simulink model "VSG_loadPR1116"  (R2015a)
settings: Solver=ode23tb  StartTime=0.0  StopTime=2  MaxStep=1e-4  MinStep=1e-7  RelTol=1e-7
InitFcn:
  | fs=1/10e3;
  | gTs=1/10e3;
libraries: powerlib x18, powerlib_meascontrol x6
settings Model: Creator=ewei  LastModifiedBy=GenkiShoo
settings DebuggingCC: UnderspecifiedInitializationDetection=Classic  MergeDetectMultiDrivingBlocksExec=none  SolverPrmCheckMsg=warning  StateNameClashWarn=warning

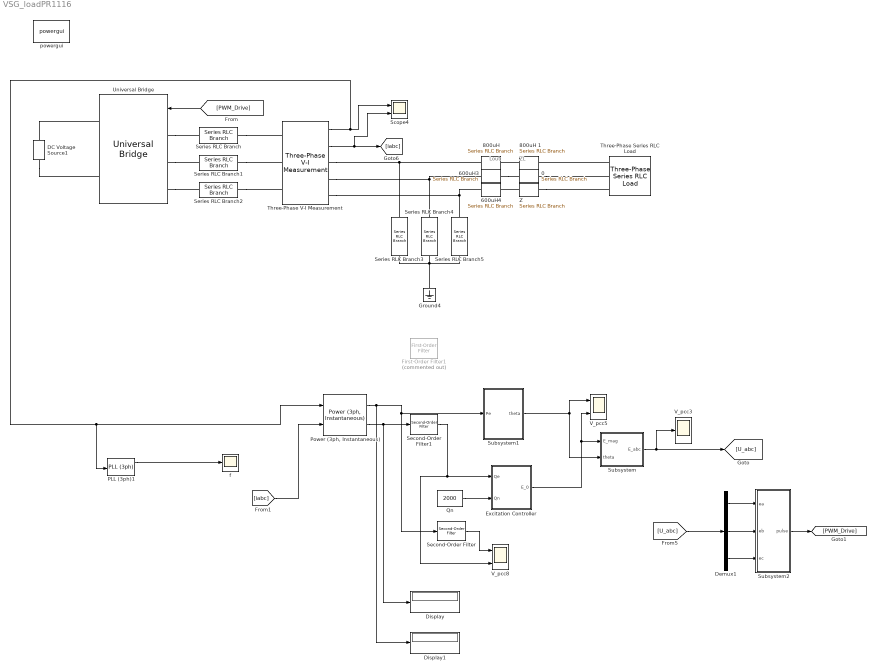
== system VSG_loadPR1116 ==
  note: ZL
  note: Lout
  0 : powerlib/Elements/Series RLC Branch  LConnTagsString=__new0  RConnTagsString=__new0  BranchType=R  Resistance=0.077+0.017i  Inductance=6e-3  SetiL0=off  InitialCurrent=0  Capacitance=[]  Setx0=off  InitialVoltage=0  Measurements=None
  600uH3 : powerlib/Elements/Series RLC Branch  LConnTagsString=__new0  RConnTagsString=__new0  BranchType=L  Resistance=0.001  Inductance=6e-3  SetiL0=off  InitialCurrent=0  Capacitance=[]  Setx0=off  InitialVoltage=0  Measurements=None
  600uH4 : powerlib/Elements/Series RLC Branch  LConnTagsString=__new0  RConnTagsString=__new0  BranchType=L  Resistance=0.001  Inductance=6e-3  SetiL0=off  InitialCurrent=0  Capacitance=[]  Setx0=off  InitialVoltage=0  Measurements=None
  "800uH " : powerlib/Elements/Series RLC Branch  LConnTagsString=__new0  RConnTagsString=__new0  BranchType=L  Resistance=0.001  Inductance=6e-3  SetiL0=off  InitialCurrent=0  Capacitance=[]  Setx0=off  InitialVoltage=0  Measurements=None
  800uH 1 : powerlib/Elements/Series RLC Branch  LConnTagsString=__new0  RConnTagsString=__new0  BranchType=R  Resistance=0.077+0.017i  Inductance=6e-3  SetiL0=off  InitialCurrent=0  Capacitance=[]  Setx0=off  InitialVoltage=0  Measurements=None
  DC Voltage Source1 : powerlib/Electrical Sources/DC Voltage Source  Amplitude=1000  Measurements=None
  Demux1 : Demux  Outputs=3
  Display : Display
  Display1 : Display
  Excitation Controller : Subsystem  mask{K=1/6000, U0=311}
  First-Order Filter1 : powerlib_meascontrol/Filters/First-Order Filter  Commented=on  FilterType=Lowpass  Tc=10e-3  Ts=0  Initialize=on  Vac_Init=[0, 0, 52]  Vdc_Init=0  PlotResponse=off  FreqRange="[0,  200,  1]"
  Ground4 : powerlib/Elements/Ground  LConnTagsString=a
  PLL (3ph)1 : powerlib_meascontrol/PLL/PLL (3ph)  Fmin=45  Par_Init=[0, 50]  ParK=[180, 3200, 1]  TcD=1e-4  MaxRateChangeFreq=12  FilterCutOffFreq=25  Ts=0  AGC=on
  "Power (3ph, Instantaneous)" : powerlib_meascontrol/Measurements/Power (3ph, Instantaneous)
  Qn : Constant  Value=2000
  Scope4 : Scope  NumInputPorts=2
      settings: YMin=-550~-150  YMax=550~125  SaveName=ScopeData8
  Second-Order Filter : powerlib_meascontrol/Filters/Second-Order Filter  FilterType=Lowpass  Fo=20  Zeta=0.707  Ts=0  Initialize=off  Vac_Init="[0,  0,  60]"  Vdc_Init=0  PlotResponse=off  FreqRange=[0, 500, 1]
  Second-Order Filter1 : powerlib_meascontrol/Filters/Second-Order Filter  FilterType=Lowpass  Fo=20  Zeta=0.707  Ts=0  Initialize=off  Vac_Init="[0,  0,  60]"  Vdc_Init=0  PlotResponse=off  FreqRange=[0, 500, 1]
  Series RLC Branch : powerlib/Elements/Series RLC Branch  LConnTagsString=__new0  RConnTagsString=__new0  BranchType=RL  Resistance=0.1  Inductance=2e-3  SetiL0=off  InitialCurrent=0  Capacitance=1e-6  Setx0=off  InitialVoltage=0  Measurements=None
  Series RLC Branch1 : powerlib/Elements/Series RLC Branch  LConnTagsString=__new0  RConnTagsString=__new0  BranchType=RL  Resistance=0.1  Inductance=2e-3  SetiL0=off  InitialCurrent=0  Capacitance=1e-6  Setx0=off  InitialVoltage=0  Measurements=None
  Series RLC Branch2 : powerlib/Elements/Series RLC Branch  LConnTagsString=__new0  RConnTagsString=__new0  BranchType=RL  Resistance=0.1  Inductance=2e-3  SetiL0=off  InitialCurrent=0  Capacitance=1e-6  Setx0=off  InitialVoltage=0  Measurements=None
  Series RLC Branch3 : powerlib/Elements/Series RLC Branch  LConnTagsString=__new0  RConnTagsString=__new0  BranchType=RC  Resistance=4  Inductance=1e-3  SetiL0=off  InitialCurrent=0  Capacitance=40e-6  Setx0=off  InitialVoltage=0  Measurements=None
  Series RLC Branch4 : powerlib/Elements/Series RLC Branch  LConnTagsString=__new0  RConnTagsString=__new0  BranchType=RC  Resistance=4  Inductance=1e-3  SetiL0=off  InitialCurrent=0  Capacitance=40e-6  Setx0=off  InitialVoltage=0  Measurements=None
  Series RLC Branch5 : powerlib/Elements/Series RLC Branch  LConnTagsString=__new0  RConnTagsString=__new0  BranchType=RC  Resistance=4  Inductance=1e-3  SetiL0=off  InitialCurrent=0  Capacitance=40e-6  Setx0=off  InitialVoltage=0  Measurements=None
  Subsystem : Subsystem
  Subsystem1 : Subsystem  mask{w0=314.15, R=1/10000, Tj=400, Kd=0, P0=20000}
      mask DialogControl parameter Prompt: parameter
  Subsystem2 : Subsystem
  Three-Phase Series RLC Load : powerlib/Elements/Three-Phase Series RLC Load  LConnTagsString=A|B|C  Configuration=Y (grounded)  NominalVoltage=380  NominalFrequency=50  ActivePower=17500  InductivePower=8000  CapacitivePower=0  Measurements=Branch voltages and currents  LoadType=constant Z
  Three-Phase V-I Measurement : powerlib/Measurements/Three-Phase V-I Measurement  VoltageMeasurement=phase-to-ground  SetLabelV=off  LabelV=Vabc  Vpu=off  VpuLL=off  CurrentMeasurement=yes  SetLabelI=off  LabelI=Iabc  Ipu=off  Pbase=100e6  Vbase=500e3  OutputType=Complex  PhasorSimulation=off  PSBequivalent=0
  Universal Bridge : powerlib/Power Electronics/Universal Bridge  Arms=3  SnubberResistance=1e5  SnubberCapacitance=inf  Device=IGBT / Diodes  Ron=1e-3  Lon=0  ForwardVoltages="[  0  0  ]"  ForwardVoltage=0  GTOparameters=[ 10e-6 , 20e-6 ]  IGBTparameters=[ 1e-6 , 2e-6 ]  Measurements=None  Measurements_2=None  converterType=Rectifier
  V_pcc3 : Scope
      settings: TimeRange=0.06000000000000001  YMin=-350  YMax=300
  V_pcc5 : Scope  NumInputPorts=2
      settings: TimeRange=2  YMin=120~312.291  YMax=126.5~312.291  SaveName=ScopeData7
  V_pcc8 : Scope  NumInputPorts=2
      settings: YMin=12600~6875  YMax=13050~7350  SaveName=ScopeData9
  Z : powerlib/Elements/Series RLC Branch  LConnTagsString=__new0  RConnTagsString=__new0  BranchType=R  Resistance=0.077+0.017i  Inductance=6e-3  SetiL0=off  InitialCurrent=0  Capacitance=[]  Setx0=off  InitialVoltage=0  Measurements=None
  f : Scope
      settings: YMin=50.259  YMax=50.272  SaveName=ScopeData10
  powergui : powerlib/powergui  Priority=1  SimulationMode=Discrete  SolverType=Tustin  SampleTime=5e-6  frequency=60  SPID=on  DisableSnubberDevices=off  DisableRonSwitches=off  DisableVfSwitches=off  SwTol=0  DisplayEquations=off  Interpol=off  methode=off  Ts=0  FunctionMessages=off  echomessages=off  HookPort=off  EnableUseOfTLC=off  x0status=blocks  frequencyindice=0  Pbase=100e6  ErrMax=1e-4  Iterations=50  UnitsV=kV  UnitsW=MW  buscounter=0  RestoreLinks=warning  ResistiveCurrentMeasurement=off  Frange=[0:2:500]  Ylog=off  Xlog=on  ShowGrid=off  save=off  variable=ZData  structure=0  ZoomFFT=off  StartTime=0.0  cycles=1  DisplayStyle=1  fundamental=60  FreqAxis=off  MaxFrequency=1000  frequencyindicesteady=1  RmsSteady=1  display=off
  wires:
  [PWM_Drive] -> Universal Bridge/1
  Qn/1 -> Excitation Controller/2(Qn)
  Excitation Controller/1(E_0) -> Subsystem/1(E_mag), V_pcc5/2
  Subsystem/1(E_abc) -> V_pcc3/1, [U_abc]
  Three-Phase V-I Measurement/2 -> Scope4/2, [iabc]
  Subsystem1/1(theta) -> Subsystem/2(theta), V_pcc5/1
  Subsystem2/1(pulse) -> [PWM_Drive]
  Demux1/1 -> Subsystem2/1(ea)
  [U_abc] -> Demux1/1
  Demux1/2 -> Subsystem2/2(eb)
  Demux1/3 -> Subsystem2/3(ec)
  "Power (3ph, Instantaneous)"/1 -> Display1/1, Second-Order Filter/1, Subsystem1/1(Pe)
  "Power (3ph, Instantaneous)"/2 -> Display/1, Second-Order Filter1/1
  PLL (3ph)1/1 -> f/1
  Three-Phase V-I Measurement/1 -> "Power (3ph, Instantaneous)"/1, PLL (3ph)1/1, Scope4/1
  [iabc] -> "Power (3ph, Instantaneous)"/2
  Second-Order Filter/1 -> V_pcc8/1
  Second-Order Filter1/1 -> V_pcc8/2, Excitation Controller/1(Qe)
  connections:
  Three-Phase V-I Measurement/RConn3 -- Series RLC Branch5/RConn1 -- 600uH4/LConn1
  Three-Phase V-I Measurement/RConn2 -- Series RLC Branch4/RConn1 -- 600uH3/LConn1
  Three-Phase V-I Measurement/RConn1 -- "800uH "/LConn1 -- Series RLC Branch3/RConn1
  DC Voltage Source1/LConn1 -- Universal Bridge/RConn2
  Series RLC Branch/RConn1 -- Three-Phase V-I Measurement/LConn1
  Series RLC Branch1/RConn1 -- Three-Phase V-I Measurement/LConn2
  DC Voltage Source1/RConn1 -- Universal Bridge/RConn1
  Series RLC Branch2/RConn1 -- Three-Phase V-I Measurement/LConn3
  Series RLC Branch3/LConn1 -- Ground4/LConn1 -- Series RLC Branch5/LConn1 -- Series RLC Branch4/LConn1
  800uH 1/LConn1 -- "800uH "/RConn1
  600uH3/RConn1 -- 0/LConn1
  Z/LConn1 -- 600uH4/RConn1
  Universal Bridge/LConn2 -- Series RLC Branch1/LConn1
  Universal Bridge/LConn3 -- Series RLC Branch2/LConn1
  Universal Bridge/LConn1 -- Series RLC Branch/LConn1
  Three-Phase Series RLC Load/LConn1 -- 800uH 1/RConn1
  0/RConn1 -- Three-Phase Series RLC Load/LConn2
  Z/RConn1 -- Three-Phase Series RLC Load/LConn3

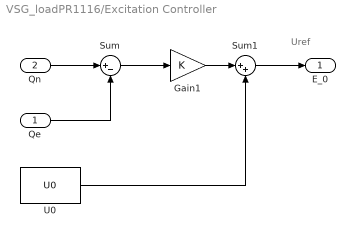
== system VSG_loadPR1116/Excitation Controller ==
  note: Uref
  Qe : Inport
  Qn : Inport  Port=2
  Gain1 : Gain  Gain=K  SaturateOnIntegerOverflow=on  OutDataTypeStr=Inherit: Same as input  ParamDataTypeStr=Inherit: Same as input
  Sum : Sum  Inputs=|+-
  Sum1 : Sum  Inputs=|++
  U0 : Constant  Value=U0  VectorParams1D=off
  E_0 : Outport
  wires:
  Qn/1 -> Sum/1
  Qe/1 -> Sum/2
  Sum/1 -> Gain1/1
  Gain1/1 -> Sum1/1
  Sum1/1 -> E_0/1
  U0/1 -> Sum1/2

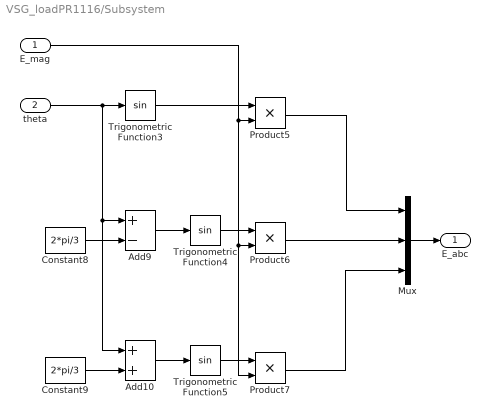
== system VSG_loadPR1116/Subsystem ==
  E_mag : Inport
  theta : Inport  Port=2
  Add10 : Sum
  Add9 : Sum  Inputs=+-
  Constant8 : Constant  Value=2*pi/3
  Constant9 : Constant  Value=2*pi/3
  Mux : Mux  Inputs=3
  Product5 : Product
  Product6 : Product
  Product7 : Product
  Trigonometric Function3 : Trigonometry
  Trigonometric Function4 : Trigonometry
  Trigonometric Function5 : Trigonometry
  E_abc : Outport
  wires:
  Constant8/1 -> Add9/2
  E_mag/1 -> Product7/2, Product6/2, Product5/2
  Add10/1 -> Trigonometric Function5/1
  theta/1 -> Trigonometric Function3/1, Add9/1, Add10/1
  Trigonometric Function5/1 -> Product7/1
  Constant9/1 -> Add10/2
  Add9/1 -> Trigonometric Function4/1
  Trigonometric Function3/1 -> Product5/1
  Trigonometric Function4/1 -> Product6/1
  Mux/1 -> E_abc/1
  Product6/1 -> Mux/2
  Product7/1 -> Mux/3
  Product5/1 -> Mux/1

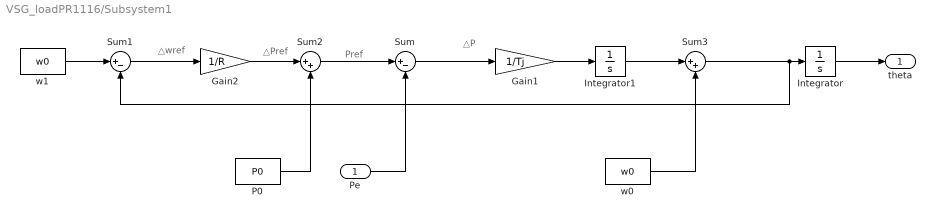
== system VSG_loadPR1116/Subsystem1 ==
  note: △P
  note: Pref
  note: △Pref
  note: △wref
  Pe : Inport
  Gain1 : Gain  Gain=1/Tj  SaturateOnIntegerOverflow=on  OutDataTypeStr=Inherit: Same as input  ParamDataTypeStr=Inherit: Same as input
  Gain2 : Gain  Gain=1/R  SaturateOnIntegerOverflow=on  OutDataTypeStr=Inherit: Same as input  ParamDataTypeStr=Inherit: Same as input
  Integrator : Integrator
  Integrator1 : Integrator
  P0 : Constant  Value=P0  VectorParams1D=off
  Sum : Sum  Inputs=|+-
  Sum1 : Sum  Inputs=|+-
  Sum2 : Sum  Inputs=|++
  Sum3 : Sum  Inputs=|++
  w0 : Constant  Value=w0  VectorParams1D=off
  w1 : Constant  Value=w0  VectorParams1D=off
  theta : Outport
  wires:
  Pe/1 -> Sum/2
  Sum/1 -> Gain1/1
  Sum2/1 -> Sum/1
  P0/1 -> Sum2/2
  Integrator/1 -> theta/1
  Gain2/1 -> Sum2/1
  w1/1 -> Sum1/1
  Sum1/1 -> Gain2/1
  Gain1/1 -> Integrator1/1
  Sum3/1 -> Sum1/2, Integrator/1
  w0/1 -> Sum3/2
  Integrator1/1 -> Sum3/1

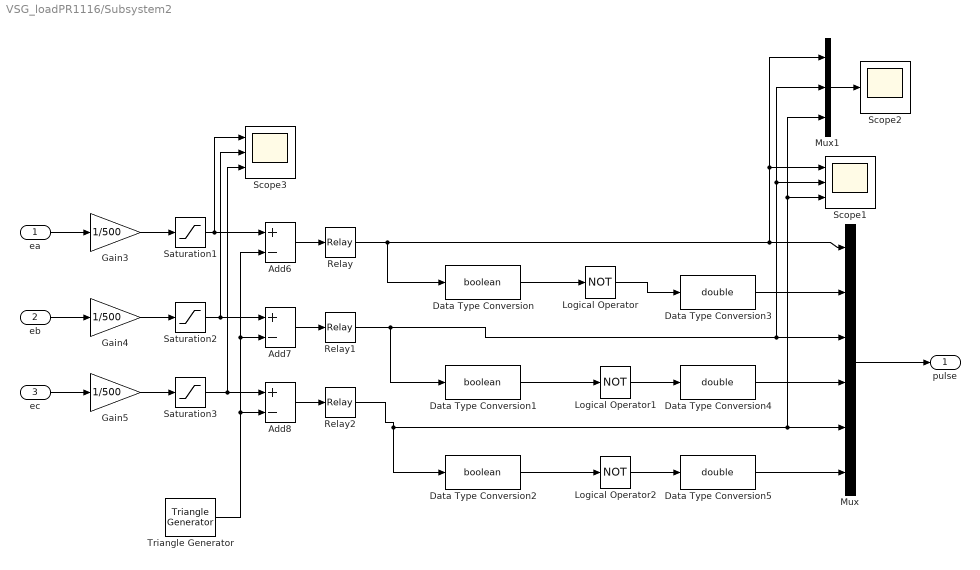
== system VSG_loadPR1116/Subsystem2 ==
  ea : Inport
  eb : Inport  Port=2
  ec : Inport  Port=3
  Add6 : Sum  Inputs=+-
  Add7 : Sum  Inputs=+-
  Add8 : Sum  Inputs=+-
  Data Type Conversion : DataTypeConversion  OutDataTypeStr=boolean
  Data Type Conversion1 : DataTypeConversion  OutDataTypeStr=boolean
  Data Type Conversion2 : DataTypeConversion  OutDataTypeStr=boolean
  Data Type Conversion3 : DataTypeConversion  OutDataTypeStr=double
  Data Type Conversion4 : DataTypeConversion  OutDataTypeStr=double
  Data Type Conversion5 : DataTypeConversion  OutDataTypeStr=double
  Gain3 : Gain  Gain=1/500
  Gain4 : Gain  Gain=1/500
  Gain5 : Gain  Gain=1/500
  Logical Operator : Logic  Operator=NOT  AllPortsSameDT=off  OutDataTypeStr=boolean
  Logical Operator1 : Logic  Operator=NOT  AllPortsSameDT=off  OutDataTypeStr=boolean
  Logical Operator2 : Logic  Operator=NOT  AllPortsSameDT=off  OutDataTypeStr=boolean
  Mux : Mux  Inputs=6
  Mux1 : Mux  Inputs=3
  Relay : Relay  OffSwitchValue=-eps
  Relay1 : Relay  OffSwitchValue=-eps
  Relay2 : Relay  OffSwitchValue=-eps
  Saturation1 : Saturate  UpperLimit=1  LowerLimit=-1
  Saturation2 : Saturate  UpperLimit=1  LowerLimit=-1
  Saturation3 : Saturate  UpperLimit=1  LowerLimit=-1
  Scope1 : Scope  NumInputPorts=3
      settings: YMin=-1.5~-1.5~-1.5  YMax=1.5~1.5~1.5  SaveName=ScopeData3
  Scope2 : Scope
      settings: YMin=-1.5  YMax=1.5  SaveName=ScopeData4
  Scope3 : Scope  NumInputPorts=3
      settings: YMin=-1.5~-1.5~-1.5  YMax=1.5~1.5~1.5  SaveName=ScopeData5
  Triangle Generator : powerlib_meascontrol/Pulse & Signal Generators/Triangle Generator  Freq=6000  Phase=0  Ts=0
  pulse : Outport
  wires:
  Triangle Generator/1 -> Add8/2, Add7/2, Add6/2
  Add6/1 -> Relay/1
  Logical Operator1/1 -> Data Type Conversion4/1
  Add8/1 -> Relay2/1
  Relay1/1 -> Data Type Conversion1/1, Mux1/2, Scope1/2, Mux/3
  Add7/1 -> Relay1/1
  Logical Operator/1 -> Data Type Conversion3/1
  Relay/1 -> Data Type Conversion/1, Scope1/1, Mux1/1, Mux/1
  Mux/1 -> pulse/1
  Logical Operator2/1 -> Data Type Conversion5/1
  Relay2/1 -> Data Type Conversion2/1, Mux1/3, Scope1/3, Mux/5
  Data Type Conversion/1 -> Logical Operator/1
  Data Type Conversion1/1 -> Logical Operator1/1
  Data Type Conversion2/1 -> Logical Operator2/1
  Data Type Conversion3/1 -> Mux/2
  Data Type Conversion4/1 -> Mux/4
  Data Type Conversion5/1 -> Mux/6
  Mux1/1 -> Scope2/1
  Saturation3/1 -> Scope3/3, Add8/1
  Saturation2/1 -> Scope3/2, Add7/1
  Saturation1/1 -> Scope3/1, Add6/1
  ea/1 -> Gain3/1
  Gain3/1 -> Saturation1/1
  eb/1 -> Gain4/1
  Gain4/1 -> Saturation2/1
  Gain5/1 -> Saturation3/1
  ec/1 -> Gain5/1
